simulink model "temp_filter"  (R2022b)
settings: Solver=VariableStepAuto  StartTime=0.0  StopTime=10.0  RelTol=1e-3
values from neighbouring files (symbols this model uses):
  f_T = time(2)-time(1)    [temperature_test.m]
  variance_T = max(difference)    [temperature_test.m]
libraries: dspstat3 x1
settings Model: Creator=aceao  LastModifiedBy=aceao

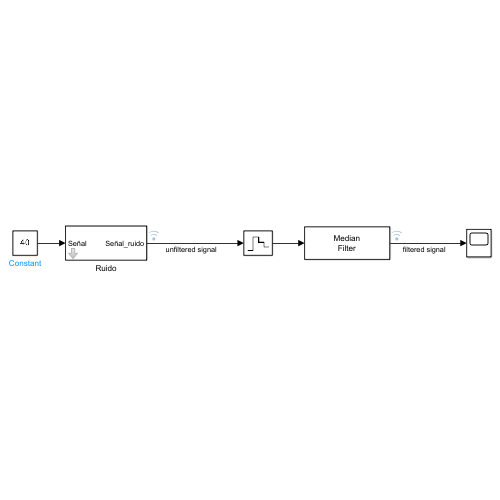
[thumbnail: Simulink's stored preview of the top-level diagram]
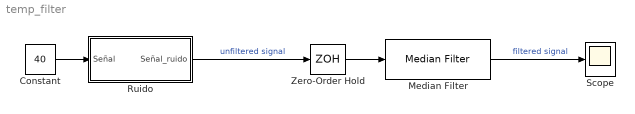
== system temp_filter ==
  Constant : Constant  Value=40
  Median Filter : dspstat3/Median Filter  WindowLength=30  SimulateUsing=Interpreted execution
      settings: LibrarySourceBlock=|
      | dspfdesign/Median
      | Filter
  Ruido : Subsystem  mask{M=0, V=variance_T, T=f_T}
      mask prompts: M "Media"; V "Varianza"; T "Periodo"
      mask DialogControl Ruido Prompt: Ruido
      mask DialogControl DescTextVar Prompt: Añade ruido gaussiano
  Scope : Scope
  Zero-Order Hold : ZeroOrderHold  SampleTime=f_T
  wires:
  Ruido/1(Señal_ruido) -> Zero-Order Hold/1  "unfiltered signal"
  Median Filter/1 -> Scope/1  "filtered signal"
  Constant/1 -> Ruido/1(Señal)
  Zero-Order Hold/1 -> Median Filter/1

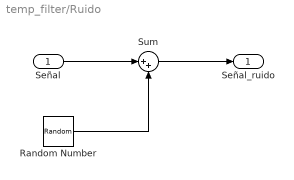
== system temp_filter/Ruido ==
  Señal : Inport
  Random Number : RandomNumber  Mean=M  Variance=V  Seed=3  SampleTime=T
  Sum : Sum  Inputs=|++
  Señal_ruido : Outport
  wires:
  Random Number/1 -> Sum/2
  Señal/1 -> Sum/1
  Sum/1 -> Señal_ruido/1
